simulink model "sysgenQAM16"  (Simulink 7.3)
settings: Solver=ode45  StartTime=0.0  StopTime=5000  RelTol=1e-3
PreLoadFcn:
  | xlrequire('PreLoadFcn')
values from neighbouring files (symbols this model uses):
  hh = hh1/max(hh1)    [sysgenCostasLoop_PreLoadFcn.m]
  j = find(xLabel==')')    [sdspfscope2_r13.m]
  k = (k-1)*3+2    [sdspfscope2_r13.m]
  mu = xfix({xlSigned, 18, 15, xlRound, xlSaturate}, mu)    [lmsErr.m]
undefined symbols (not defined in the file or in its folder): chan, k_i0, k_p0, xlipgetpartsetting, xlsfunxy
libraries: xbsIndex_r4 x263, dspmlti4 x2, dspsigops x2, dspbuff3 x1, xbsCopyrightNotice_r4 x1, dspobslib x1, simulink x1, dspsnks4 x1
(part 2 of 4)

== system sysgenQAM16/Carrier Recovery/DPLL Loop Filter ==
  phs_err : Inport  OutDataType=sfix(16)  OutScaling=2^0
  KI : xbsIndex_r4/Constant  Priority=5  arith_type=Signed (2's comp)  const=k_i0  n_bits=16  bin_pt=15  explicit_period=on  period=4  equ=P=C  opselect=C  inp2=PCIN>>17  opr=+  inp1=P  carry=CIN  dbl_ovrd=off  block_type=constant
      settings: block_version=VER_STRING_GOES_HERE
  KP : xbsIndex_r4/Constant  Priority=5  arith_type=Signed (2's comp)  const=k_p0  n_bits=16  bin_pt=15  explicit_period=on  period=4  equ=P=C  opselect=C  inp2=PCIN>>17  opr=+  inp1=P  carry=CIN  dbl_ovrd=off  block_type=constant
      settings: block_version=VER_STRING_GOES_HERE
  MPY KI : xbsIndex_r4/Mult  precision=User Defined  arith_type="Signed  (2's comp)"  n_bits=32  bin_pt=28  quantization=Truncate  overflow=Wrap  en=off  latency=0  dbl_ovrd=off  use_behavioral_HDL=off  opt=Speed  use_embedded=on  optimum_pipeline=off  pipeline=off  use_rpm=off  placement_style=Rectangular shape  block_type=mult
      settings: infoedit=Multiplies two values.<P><P>Hardware notes: To use the internal pipeline stage of the dedicated multiplier you must select 'Pipeline to Greatest Extent Possible'.  xl_area=[11 0 0 22 0 2 0]  block_version=VER_STRING_GOES_HERE
  MPY KP : xbsIndex_r4/Mult  precision=User Defined  arith_type="Signed  (2's comp)"  n_bits=32  bin_pt=28  quantization=Truncate  overflow=Wrap  en=off  latency=0  dbl_ovrd=off  use_behavioral_HDL=off  opt=Speed  use_embedded=on  optimum_pipeline=off  pipeline=off  use_rpm=off  placement_style=Rectangular shape  block_type=mult
      settings: infoedit=Multiplies two values.<P><P>Hardware notes: To use the internal pipeline stage of the dedicated multiplier you must select 'Pipeline to Greatest Extent Possible'.  xl_area=[11 0 0 22 0 2 0]  block_version=VER_STRING_GOES_HERE
  addsub : xbsIndex_r4/AddSub  mode=Addition  use_carryin=off  use_carryout=off  en=off  latency=0  precision=User Defined  arith_type=Unsigned  n_bits=10  bin_pt=10  quantization=Truncate  overflow=Wrap  dbl_ovrd=off  use_behavioral_HDL=on  hw_selection=Fabric  pipelined=off  use_rpm=off  block_type=addsub
      settings: xl_area=[14 0 0 28 0 0 0]  block_version=VER_STRING_GOES_HERE
  addsub1 : xbsIndex_r4/AddSub  mode=Addition  use_carryin=off  use_carryout=off  en=off  latency=0  precision=User Defined  arith_type="Signed  (2's comp)"  n_bits=32  bin_pt=28  quantization="Round  (unbiased: +/- Inf)"  overflow=Wrap  dbl_ovrd=off  use_behavioral_HDL=on  hw_selection=Fabric  pipelined=off  use_rpm=off  block_type=addsub
      settings: xl_area=[16 0 0 32 0 0 0]  block_version=VER_STRING_GOES_HERE
  register : xbsIndex_r4/Register  init=0  rst=off  en=off  dbl_ovrd=off  block_type=register
      settings: xl_area=[16 32 0 0 0 0 0]  block_version=VER_STRING_GOES_HERE
  y : Outport  OutDataType=sfix(16)  OutScaling=2^0
  wires:
  KI/1 -> MPY KI/2
  KP/1 -> MPY KP/2
  MPY KI/1 -> addsub1/1
  phs_err/1 -> MPY KI/1, MPY KP/1
  register/1 -> addsub1/2
  addsub1/1 -> addsub/2, register/1
  MPY KP/1 -> addsub/1
  addsub/1 -> y/1

== system sysgenQAM16/Carrier Recovery/Phase Detector ==
  note: The slicer circuit consistis primarily of several
      | comparators and a small look-up table.
  note: The arctangent operation is performed using
      | a custom CORDIC processor.
  I_in : Inport  OutDataType=sfix(16)  OutScaling=2^0
  Q_in : Inport  Port=2  OutDataType=sfix(16)  OutScaling=2^0
  Constant : xbsIndex_r4/Constant  arith_type=Signed (2's comp)  const=0  n_bits=1  bin_pt=0  explicit_period=off  period=1  equ=P=C  opselect=C  inp2=PCIN>>17  opr=+  inp1=P  carry=CIN  dbl_ovrd=off  block_type=constant
      settings: block_version=VER_STRING_GOES_HERE
  Cordic : Subsystem
  NegB_Cmplx Mult : Subsystem
  Slicer : Subsystem
  Terminator : Terminator
  Terminator1 : Terminator
  det_I : Outport  OutDataType=sfix(16)  OutScaling=2^0
  det_Q : Outport  Port=2  OutDataType=sfix(16)  OutScaling=2^0
  phs_err : Outport  Port=3  OutDataType=sfix(16)  OutScaling=2^0
  wires:
  NegB_Cmplx Mult/1(p_r) -> Cordic/1(x)
  Cordic/3(z_n) -> phs_err/1
  Constant/1 -> Cordic/3(z)
  Cordic/1(x_n) -> Terminator/1
  Cordic/2(y_n) -> Terminator1/1
  NegB_Cmplx Mult/2(p_i) -> Cordic/2(y)
  Slicer/2(det_Q) -> NegB_Cmplx Mult/2(a_i), det_Q/1
  Slicer/1(det_ I) -> NegB_Cmplx Mult/1(a_r), det_I/1
  Q_in/1 -> Slicer/2(Q_in), NegB_Cmplx Mult/4(b_i)
  I_in/1 -> Slicer/1(I_in), NegB_Cmplx Mult/3(b_r)

== system sysgenQAM16/Channel/Channel ==
  x_n : Inport  OutDataType=sfix(16)  OutScaling=2^0
  Channel Response : Subsystem
  y_n : Outport  OutDataType=sfix(16)  OutScaling=2^0
  wires:
  Channel Response/1(y_n) -> y_n/1
  x_n/1 -> Channel Response/1(x_n)

== system sysgenQAM16/Channel/Channel1 ==
  x_n : Inport  OutDataType=sfix(16)  OutScaling=2^0
  Channel Response : Subsystem
  y_n : Outport  OutDataType=sfix(16)  OutScaling=2^0
  wires:
  Channel Response/1(y_n) -> y_n/1
  x_n/1 -> Channel Response/1(x_n)

== system sysgenQAM16/Doppler/TX Doppler ==
  In1 : Inport  OutDataType=sfix(16)  OutScaling=2^0
  Sum5 : Sum  Inputs=|++  OutDataType=sfix(16)  OutScaling=2^0  SaturateOnIntegerOverflow=on  InputSameDT=on  OutDataTypeStr=Inherit: Same as first input
  Trigonometric Function1 : Trigonometry  Operator=cos
  Trigonometric Function2 : Trigonometry
  Unit Delay2 : UnitDelay
  c2 : Gain  Gain=2*pi  ParameterDataType=sfix(16)  ParameterScaling=2^0  OutDataType=sfix(16)  OutScaling=2^0  SaturateOnIntegerOverflow=on  OutDataTypeStr=Inherit: Same as input  ParamDataTypeStr=Inherit: Same as input
  c3 : Gain  ParameterDataType=sfix(16)  ParameterScaling=2^0  OutDataType=sfix(16)  OutScaling=2^0  SaturateOnIntegerOverflow=on  OutDataTypeStr=Inherit: Same as input  ParamDataTypeStr=Inherit: Same as input
  Cos : Outport  OutDataType=sfix(16)  OutScaling=2^0
  Sin : Outport  Port=2  OutDataType=sfix(16)  OutScaling=2^0
  DDS Theta : Outport  Port=3  OutDataType=sfix(16)  OutScaling=2^0
  wires:
  c2/1 -> Trigonometric Function1/1, Trigonometric Function2/1, DDS Theta/1
  Sum5/1 -> Unit Delay2/1
  Unit Delay2/1 -> c2/1, Sum5/2
  Trigonometric Function2/1 -> c3/1
  c3/1 -> Sin/1
  Trigonometric Function1/1 -> Cos/1
  In1/1 -> Sum5/1

== system sysgenQAM16/16-QAM Data Shaping & Interpolation/QAM16 Source/QAM16 - I ==
  Constant : Constant  Value=3  OutDataType=sfix(16)  OutScaling=2^0
  Gain : Gain  Gain=2  ParameterDataType=sfix(16)  ParameterScaling=2^0  OutDataType=sfix(16)  OutScaling=2^0  SaturateOnIntegerOverflow=on  OutDataTypeStr=Inherit: Same as input  ParamDataTypeStr=Inherit: Same as input
  Gain1 : Gain  Gain=1/3  ParameterDataType=sfix(16)  ParameterScaling=2^0  OutDataType=sfix(16)  OutScaling=2^0  SaturateOnIntegerOverflow=on  OutDataTypeStr=Inherit: Same as input  ParamDataTypeStr=Inherit: Same as input
  Random Integer Generator : Subsystem  mask{M=4, seed=11, Ts=4}
      mask prompts: M "M-ary Number"; seed "Initial seed"; Ts "Sample Time"
  Sum : Sum  Inputs=|+-  OutDataType=sfix(16)  OutScaling=2^0  SaturateOnIntegerOverflow=on  InputSameDT=on  OutDataTypeStr=Inherit: Same as first input
  I : Outport  OutDataType=sfix(16)  OutScaling=2^0
  wires:
  Gain1/1 -> I/1
  Sum/1 -> Gain1/1
  Constant/1 -> Sum/2
  Gain/1 -> Sum/1
  Random Integer Generator/1(Out1) -> Gain/1

== system sysgenQAM16/16-QAM Data Shaping & Interpolation/QAM16 Source/QAM16 -Q ==
  Constant : Constant  Value=3  OutDataType=sfix(16)  OutScaling=2^0
  Gain : Gain  Gain=2  ParameterDataType=sfix(16)  ParameterScaling=2^0  OutDataType=sfix(16)  OutScaling=2^0  SaturateOnIntegerOverflow=on  OutDataTypeStr=Inherit: Same as input  ParamDataTypeStr=Inherit: Same as input
  Gain1 : Gain  Gain=1/3  ParameterDataType=sfix(16)  ParameterScaling=2^0  OutDataType=sfix(16)  OutScaling=2^0  SaturateOnIntegerOverflow=on  OutDataTypeStr=Inherit: Same as input  ParamDataTypeStr=Inherit: Same as input
  Random Integer Generator : Subsystem  mask{M=4, seed=72, Ts=4}
      mask prompts: M "M-ary Number"; seed "Initial seed"; Ts "Sample Time"
  Sum : Sum  Inputs=|+-  OutDataType=sfix(16)  OutScaling=2^0  SaturateOnIntegerOverflow=on  InputSameDT=on  OutDataTypeStr=Inherit: Same as first input
  Q : Outport  OutDataType=sfix(16)  OutScaling=2^0
  wires:
  Gain1/1 -> Q/1
  Sum/1 -> Gain1/1
  Constant/1 -> Sum/2
  Gain/1 -> Sum/1
  Random Integer Generator/1(Out1) -> Gain/1

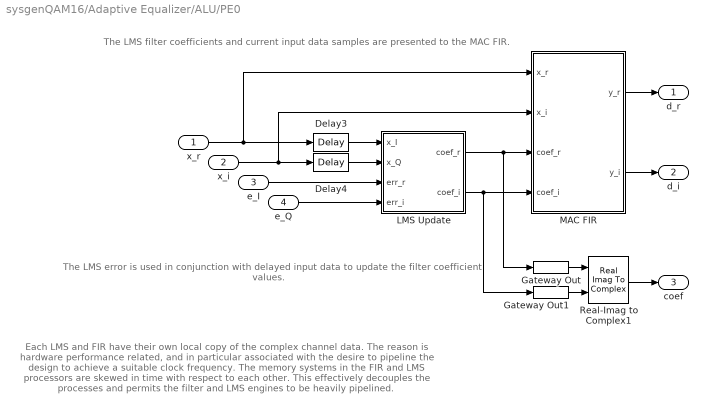
== system sysgenQAM16/Adaptive Equalizer/ALU/PE0 ==
  note: The LMS error is used in conjunction with
      | delayed input data to update the filter
      | coefficient values.
  note: The LMS filter coefficients and current input
      | data samples are presented to the MAC FIR.
  note: Each LMS and FIR have their own local copy of the complex channel data. The reason is hardware
      | performance related, and in particular associated with the desire to pipeline the design to achieve
      | a suitable clock frequency. The memory systems in the FIR and LMS processors are skewed in
      | time with respect to each other. This effectively decouples the processes and permits the filter
      | and LMS engines to be heavily pipelined.
  x_r : Inport  OutDataType=sfix(16)  OutScaling=2^0
  x_i : Inport  Port=2  OutDataType=sfix(16)  OutScaling=2^0
  e_I : Inport  Port=3  OutDataType=sfix(16)  OutScaling=2^0
  e_Q : Inport  Port=4  OutDataType=sfix(16)  OutScaling=2^0
  Delay3 : xbsIndex_r4/Delay  en=off  latency=k  dbl_ovrd=off  reg_retiming=off  block_type=delay
      settings: infoedit="Delay line having  configurable length.<P><P>Hardware notes: A delay line is a chain, each link of which is an SRL16 followed by a flip-flop. If register retiming is enabled, the delay line is a chain of flip-flops."  xl_area=[8 16 0 16 0 0 0]  block_version=VER_STRING_GOES_HERE
  Delay4 : xbsIndex_r4/Delay  en=off  latency=k  dbl_ovrd=off  reg_retiming=off  block_type=delay
      settings: infoedit="Delay line having  configurable length.<P><P>Hardware notes: A delay line is a chain, each link of which is an SRL16 followed by a flip-flop. If register retiming is enabled, the delay line is a chain of flip-flops."  xl_area=[8 16 0 16 0 0 0]  block_version=VER_STRING_GOES_HERE
  Gateway Out : xbsIndex_r4/Gateway Out  hdl_port=off  timing_constraint=None  locs_specified=off  LOCs={}  block_type=gatewayout
      settings: infoedit="Gateway out block.  Converts Xilinx fixed point inputs into ouputs of type Simulink integer, double, or fixed point.<P><P>Hardware notes:  In hardware these blocks become top level output ports or are discarded, depending on how they are configured."  xl_area=[0 0 0 0 0 0 0]  block_version=VER_STRING_GOES_HERE
  Gateway Out1 : xbsIndex_r4/Gateway Out  hdl_port=off  timing_constraint=None  locs_specified=off  LOCs={}  block_type=gatewayout
      settings: infoedit="Gateway out block.  Converts Xilinx fixed point inputs into ouputs of type Simulink integer, double, or fixed point.<P><P>Hardware notes:  In hardware these blocks become top level output ports or are discarded, depending on how they are configured."  xl_area=[0 0 0 0 0 0 0]  block_version=VER_STRING_GOES_HERE
  LMS Update : Subsystem
  MAC FIR : Subsystem
  Real-Imag to Complex1 : RealImagToComplex
  d_r : Outport  OutDataType=sfix(16)  OutScaling=2^0
  d_i : Outport  Port=2  OutDataType=sfix(16)  OutScaling=2^0
  coef : Outport  Port=3  OutDataType=sfix(16)  OutScaling=2^0
  wires:
  x_r/1 -> Delay3/1, MAC FIR/1(x_r)
  x_i/1 -> Delay4/1, MAC FIR/2(x_i)
  e_I/1 -> LMS Update/3(err_r)
  e_Q/1 -> LMS Update/4(err_i)
  Delay3/1 -> LMS Update/1(x_I)
  Delay4/1 -> LMS Update/2(x_Q)
  MAC FIR/1(y_r) -> d_r/1
  MAC FIR/2(y_i) -> d_i/1
  Gateway Out/1 -> Real-Imag to Complex1/1
  Gateway Out1/1 -> Real-Imag to Complex1/2
  Real-Imag to Complex1/1 -> coef/1
  LMS Update/2(coef_i) -> MAC FIR/4(coef_i), Gateway Out1/1
  LMS Update/1(coef_r) -> MAC FIR/3(coef_r), Gateway Out/1

== system sysgenQAM16/Adaptive Equalizer/ALU/PE1 ==
  x_r : Inport  OutDataType=sfix(16)  OutScaling=2^0
  x_i : Inport  Port=2  OutDataType=sfix(16)  OutScaling=2^0
  e_I : Inport  Port=3  OutDataType=sfix(16)  OutScaling=2^0
  e_Q : Inport  Port=4  OutDataType=sfix(16)  OutScaling=2^0
  Delay1 : xbsIndex_r4/Delay  en=off  latency=k  dbl_ovrd=off  reg_retiming=off  block_type=delay
      settings: infoedit="Delay line having  configurable length.<P><P>Hardware notes: A delay line is a chain, each link of which is an SRL16 followed by a flip-flop. If register retiming is enabled, the delay line is a chain of flip-flops."  xl_area=[8 16 0 16 0 0 0]  block_version=VER_STRING_GOES_HERE
  Delay2 : xbsIndex_r4/Delay  en=off  latency=k  dbl_ovrd=off  reg_retiming=off  block_type=delay
      settings: infoedit="Delay line having  configurable length.<P><P>Hardware notes: A delay line is a chain, each link of which is an SRL16 followed by a flip-flop. If register retiming is enabled, the delay line is a chain of flip-flops."  xl_area=[8 16 0 16 0 0 0]  block_version=VER_STRING_GOES_HERE
  Gateway Out2 : xbsIndex_r4/Gateway Out  hdl_port=off  timing_constraint=None  locs_specified=off  LOCs={}  block_type=gatewayout
      settings: infoedit="Gateway out block.  Converts Xilinx fixed point inputs into ouputs of type Simulink integer, double, or fixed point.<P><P>Hardware notes:  In hardware these blocks become top level output ports or are discarded, depending on how they are configured."  xl_area=[0 0 0 0 0 0 0]  block_version=VER_STRING_GOES_HERE
  Gateway Out3 : xbsIndex_r4/Gateway Out  hdl_port=off  timing_constraint=None  locs_specified=off  LOCs={}  block_type=gatewayout
      settings: infoedit="Gateway out block.  Converts Xilinx fixed point inputs into ouputs of type Simulink integer, double, or fixed point.<P><P>Hardware notes:  In hardware these blocks become top level output ports or are discarded, depending on how they are configured."  xl_area=[0 0 0 0 0 0 0]  block_version=VER_STRING_GOES_HERE
  LMS Update : Subsystem
  MAC FIR : Subsystem
  Real-Imag to Complex2 : RealImagToComplex
  d_r : Outport  OutDataType=sfix(16)  OutScaling=2^0
  d_i : Outport  Port=2  OutDataType=sfix(16)  OutScaling=2^0
  coef : Outport  Port=3  OutDataType=sfix(16)  OutScaling=2^0
  wires:
  Gateway Out2/1 -> Real-Imag to Complex2/1
  Gateway Out3/1 -> Real-Imag to Complex2/2
  Real-Imag to Complex2/1 -> coef/1
  Delay2/1 -> LMS Update/2(x_Q)
  Delay1/1 -> LMS Update/1(x_I)
  LMS Update/1(coef_r) -> MAC FIR/3(coef_r), Gateway Out2/1
  LMS Update/2(coef_i) -> MAC FIR/4(coef_i), Gateway Out3/1
  MAC FIR/1(y_r) -> d_r/1
  MAC FIR/2(y_i) -> d_i/1
  e_Q/1 -> LMS Update/4(err_i)
  e_I/1 -> LMS Update/3(err_r)
  x_i/1 -> Delay2/1, MAC FIR/2(x_i)
  x_r/1 -> Delay1/1, MAC FIR/1(x_r)

== system sysgenQAM16/Carrier Recovery/Phase Detector/Cordic ==
  x : Inport  OutDataType=sfix(16)  OutScaling=2^0
  y : Inport  Port=2  OutDataType=sfix(16)  OutScaling=2^0
  z : Inport  Port=3  OutDataType=sfix(16)  OutScaling=2^0
  Cordic Fine Angle PE : Subsystem
  Quadrant  Correct : Subsystem
  Quadrant  Map : Subsystem
  x_n : Outport  OutDataType=sfix(16)  OutScaling=2^0
  y_n : Outport  Port=2  OutDataType=sfix(16)  OutScaling=2^0
  z_n : Outport  Port=3  OutDataType=sfix(16)  OutScaling=2^0
  wires:
  Cordic Fine Angle PE/1(x_n) -> x_n/1
  Cordic Fine Angle PE/2(y_n) -> y_n/1
  Cordic Fine Angle PE/3(z_n) -> Quadrant  Correct/1(z_in)
  y/1 -> Quadrant  Map/2(y)
  x/1 -> Quadrant  Map/1(x)
  Quadrant  Map/2(y_map) -> Cordic Fine Angle PE/2(y_0)
  Quadrant  Map/1(x_map) -> Cordic Fine Angle PE/1(x_0)
  Quadrant  Correct/1(z_out) -> z_n/1
  Quadrant  Map/4(z_mux_sel) -> Quadrant  Correct/3(z_mux_sel)
  Quadrant  Map/3(" PI:2_add:sub") -> Quadrant  Correct/2(pi:2_add:sub)
  z/1 -> Cordic Fine Angle PE/3(z_0)

== system sysgenQAM16/Carrier Recovery/Phase Detector/NegB_Cmplx Mult ==
  a_r : Inport  OutDataType=sfix(16)  OutScaling=2^0
  a_i : Inport  Port=2  OutDataType=sfix(16)  OutScaling=2^0
  b_r : Inport  Port=3  OutDataType=sfix(16)  OutScaling=2^0
  b_i : Inport  Port=4  OutDataType=sfix(16)  OutScaling=2^0
  AddSub : xbsIndex_r4/AddSub  mode=Addition  use_carryin=off  use_carryout=off  en=off  latency=0  precision=User Defined  arith_type="Signed  (2's comp)"  n_bits=lms_mult_post_add_ni  bin_pt=lms_mult_post_add_nf  quantization=Truncate  overflow=Wrap  dbl_ovrd=off  use_behavioral_HDL=on  hw_selection=Fabric  pipelined=off  use_rpm=on  block_type=addsub
      settings: xl_area=[18 0 0 36 0 0 0]  block_version=VER_STRING_GOES_HERE
  AddSub1 : xbsIndex_r4/AddSub  mode=Subtraction  use_carryin=off  use_carryout=off  en=off  latency=0  precision=User Defined  arith_type="Signed  (2's comp)"  n_bits=lms_mult_post_add_ni  bin_pt=lms_mult_post_add_nf  quantization=Truncate  overflow=Wrap  dbl_ovrd=off  use_behavioral_HDL=on  hw_selection=Fabric  pipelined=off  use_rpm=on  block_type=addsub
      settings: xl_area=[18 0 0 36 0 0 0]  block_version=VER_STRING_GOES_HERE
  Mult{1..4} (4 alike) : xbsIndex_r4/Mult  precision=User Defined  arith_type="Signed  (2's comp)"  n_bits=lms_mult_ni  bin_pt=lms_mult_nf  quantization=Truncate  overflow=Wrap  en=off  latency=0  dbl_ovrd=off  use_behavioral_HDL=off  opt=Speed  use_embedded=on  optimum_pipeline=off  pipeline=off  use_rpm=on  placement_style=Rectangular shape  block_type=mult
      settings: infoedit=Multiplies two values.<P><P>Hardware notes: To use the internal pipeline stage of the dedicated multiplier you must select 'Pipeline to Greatest Extent Possible'.  xl_area=[69 0 0 136 0 3 0]  block_version=VER_STRING_GOES_HERE
  p_r : Outport  OutDataType=sfix(16)  OutScaling=2^0
  p_i : Outport  Port=2  OutDataType=sfix(16)  OutScaling=2^0
  wires:
  Mult4/1 -> AddSub/1
  a_i/1 -> Mult1/1, Mult3/2
  b_r/1 -> Mult4/2, Mult3/1
  b_i/1 -> Mult1/2, Mult2/2
  a_r/1 -> Mult4/1, Mult2/1
  Mult1/1 -> AddSub/2
  Mult2/1 -> AddSub1/1
  Mult3/1 -> AddSub1/2
  AddSub/1 -> p_r/1
  AddSub1/1 -> p_i/1

== system sysgenQAM16/Carrier Recovery/Phase Detector/Slicer ==
  I_in : Inport  OutDataType=sfix(16)  OutScaling=2^0
  Q_in : Inport  Port=2  OutDataType=sfix(16)  OutScaling=2^0
  I Map : Subsystem
  Q Map : Subsystem
  det_ I : Outport  OutDataType=sfix(16)  OutScaling=2^0
  det_Q : Outport  Port=2  OutDataType=sfix(16)  OutScaling=2^0
  wires:
  Q Map/1(det) -> det_Q/1
  I Map/1(det) -> det_ I/1
  I_in/1 -> I Map/1(x_n)
  Q_in/1 -> Q Map/1(x_n)

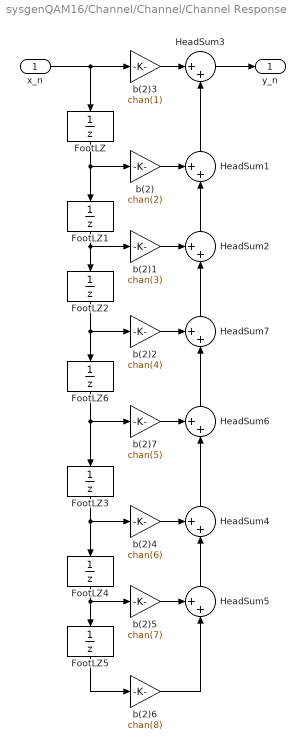
== system sysgenQAM16/Channel/Channel/Channel Response ==
  x_n : Inport  OutDataType=sfix(16)  OutScaling=2^0
  FootLZ : UnitDelay
  FootLZ{1..2,4..6} (5 alike) : UnitDelay  SampleTime=-1
  FootLZ3 : UnitDelay
  HeadSum{1..2,4..7} (6 alike) : Sum  Inputs=++|  OutDataType=sfix(16)  OutScaling=2^0  SaturateOnIntegerOverflow=on  InputSameDT=on  OutDataTypeStr=Inherit: Same as first input
  HeadSum3 : Sum  Inputs=|++  OutDataType=sfix(16)  OutScaling=2^0  SaturateOnIntegerOverflow=on  InputSameDT=on  OutDataTypeStr=Inherit: Same as first input
  b(2) : Gain  Gain=chan(2)  ParameterDataType=sfix(16)  ParameterScaling=2^0  OutDataType=sfix(16)  OutScaling=2^0  SaturateOnIntegerOverflow=on  OutDataTypeStr=Inherit: Same as input  ParamDataTypeStr=Inherit: Same as input
  b(2)1 : Gain  Gain=chan(3)  ParameterDataType=sfix(16)  ParameterScaling=2^0  OutDataType=sfix(16)  OutScaling=2^0  SaturateOnIntegerOverflow=on  OutDataTypeStr=Inherit: Same as input  ParamDataTypeStr=Inherit: Same as input
  b(2)2 : Gain  Gain=chan(4)  ParameterDataType=sfix(16)  ParameterScaling=2^0  OutDataType=sfix(16)  OutScaling=2^0  SaturateOnIntegerOverflow=on  OutDataTypeStr=Inherit: Same as input  ParamDataTypeStr=Inherit: Same as input
  b(2)3 : Gain  Gain=chan(1)  ParameterDataType=sfix(16)  ParameterScaling=2^0  OutDataType=sfix(16)  OutScaling=2^0  SaturateOnIntegerOverflow=on  OutDataTypeStr=Inherit: Same as input  ParamDataTypeStr=Inherit: Same as input
  b(2)4 : Gain  Gain=chan(6)  ParameterDataType=sfix(16)  ParameterScaling=2^0  OutDataType=sfix(16)  OutScaling=2^0  SaturateOnIntegerOverflow=on  OutDataTypeStr=Inherit: Same as input  ParamDataTypeStr=Inherit: Same as input
  b(2)5 : Gain  Gain=chan(7)  ParameterDataType=sfix(16)  ParameterScaling=2^0  OutDataType=sfix(16)  OutScaling=2^0  SaturateOnIntegerOverflow=on  OutDataTypeStr=Inherit: Same as input  ParamDataTypeStr=Inherit: Same as input
  b(2)6 : Gain  Gain=chan(8)  ParameterDataType=sfix(16)  ParameterScaling=2^0  OutDataType=sfix(16)  OutScaling=2^0  SaturateOnIntegerOverflow=on  OutDataTypeStr=Inherit: Same as input  ParamDataTypeStr=Inherit: Same as input
  b(2)7 : Gain  Gain=chan(5)  ParameterDataType=sfix(16)  ParameterScaling=2^0  OutDataType=sfix(16)  OutScaling=2^0  SaturateOnIntegerOverflow=on  OutDataTypeStr=Inherit: Same as input  ParamDataTypeStr=Inherit: Same as input
  y_n : Outport  OutDataType=sfix(16)  OutScaling=2^0
  wires:
  HeadSum3/1 -> y_n/1
  HeadSum1/1 -> HeadSum3/2
  b(2)3/1 -> HeadSum3/1
  x_n/1 -> b(2)3/1, FootLZ/1
  HeadSum2/1 -> HeadSum1/2
  b(2)1/1 -> HeadSum2/1
  b(2)/1 -> HeadSum1/1
  FootLZ1/1 -> b(2)1/1, FootLZ2/1
  FootLZ/1 -> FootLZ1/1, b(2)/1
  FootLZ2/1 -> b(2)2/1, FootLZ6/1
  b(2)7/1 -> HeadSum6/1
  b(2)6/1 -> HeadSum5/2
  HeadSum5/1 -> HeadSum4/2
  b(2)5/1 -> HeadSum5/1
  b(2)4/1 -> HeadSum4/1
  FootLZ5/1 -> b(2)6/1
  FootLZ4/1 -> b(2)5/1, FootLZ5/1
  FootLZ3/1 -> FootLZ4/1, b(2)4/1
  FootLZ6/1 -> b(2)7/1, FootLZ3/1
  b(2)2/1 -> HeadSum7/1
  HeadSum7/1 -> HeadSum2/2
  HeadSum4/1 -> HeadSum6/2
  HeadSum6/1 -> HeadSum7/2

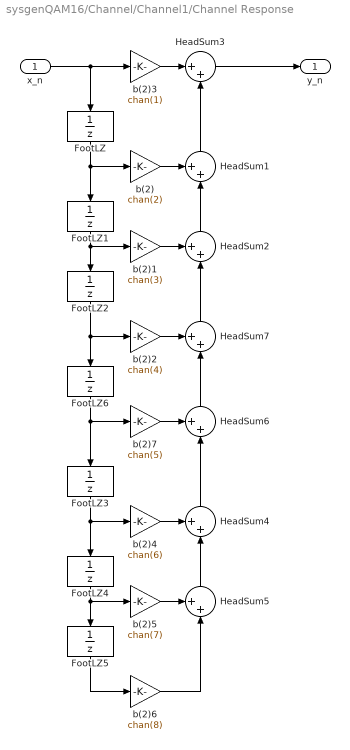
== system sysgenQAM16/Channel/Channel1/Channel Response ==
  x_n : Inport  OutDataType=sfix(16)  OutScaling=2^0
  FootLZ : UnitDelay
  FootLZ{1..2,4..6} (5 alike) : UnitDelay  SampleTime=-1
  FootLZ3 : UnitDelay
  HeadSum{1..2,4..7} (6 alike) : Sum  Inputs=++|  OutDataType=sfix(16)  OutScaling=2^0  SaturateOnIntegerOverflow=on  InputSameDT=on  OutDataTypeStr=Inherit: Same as first input
  HeadSum3 : Sum  Inputs=|++  OutDataType=sfix(16)  OutScaling=2^0  SaturateOnIntegerOverflow=on  InputSameDT=on  OutDataTypeStr=Inherit: Same as first input
  b(2) : Gain  Gain=chan(2)  ParameterDataType=sfix(16)  ParameterScaling=2^0  OutDataType=sfix(16)  OutScaling=2^0  SaturateOnIntegerOverflow=on  OutDataTypeStr=Inherit: Same as input  ParamDataTypeStr=Inherit: Same as input
  b(2)1 : Gain  Gain=chan(3)  ParameterDataType=sfix(16)  ParameterScaling=2^0  OutDataType=sfix(16)  OutScaling=2^0  SaturateOnIntegerOverflow=on  OutDataTypeStr=Inherit: Same as input  ParamDataTypeStr=Inherit: Same as input
  b(2)2 : Gain  Gain=chan(4)  ParameterDataType=sfix(16)  ParameterScaling=2^0  OutDataType=sfix(16)  OutScaling=2^0  SaturateOnIntegerOverflow=on  OutDataTypeStr=Inherit: Same as input  ParamDataTypeStr=Inherit: Same as input
  b(2)3 : Gain  Gain=chan(1)  ParameterDataType=sfix(16)  ParameterScaling=2^0  OutDataType=sfix(16)  OutScaling=2^0  SaturateOnIntegerOverflow=on  OutDataTypeStr=Inherit: Same as input  ParamDataTypeStr=Inherit: Same as input
  b(2)4 : Gain  Gain=chan(6)  ParameterDataType=sfix(16)  ParameterScaling=2^0  OutDataType=sfix(16)  OutScaling=2^0  SaturateOnIntegerOverflow=on  OutDataTypeStr=Inherit: Same as input  ParamDataTypeStr=Inherit: Same as input
  b(2)5 : Gain  Gain=chan(7)  ParameterDataType=sfix(16)  ParameterScaling=2^0  OutDataType=sfix(16)  OutScaling=2^0  SaturateOnIntegerOverflow=on  OutDataTypeStr=Inherit: Same as input  ParamDataTypeStr=Inherit: Same as input
  b(2)6 : Gain  Gain=chan(8)  ParameterDataType=sfix(16)  ParameterScaling=2^0  OutDataType=sfix(16)  OutScaling=2^0  SaturateOnIntegerOverflow=on  OutDataTypeStr=Inherit: Same as input  ParamDataTypeStr=Inherit: Same as input
  b(2)7 : Gain  Gain=chan(5)  ParameterDataType=sfix(16)  ParameterScaling=2^0  OutDataType=sfix(16)  OutScaling=2^0  SaturateOnIntegerOverflow=on  OutDataTypeStr=Inherit: Same as input  ParamDataTypeStr=Inherit: Same as input
  y_n : Outport  OutDataType=sfix(16)  OutScaling=2^0
  wires:
  HeadSum3/1 -> y_n/1
  HeadSum1/1 -> HeadSum3/2
  b(2)3/1 -> HeadSum3/1
  x_n/1 -> b(2)3/1, FootLZ/1
  HeadSum2/1 -> HeadSum1/2
  b(2)1/1 -> HeadSum2/1
  b(2)/1 -> HeadSum1/1
  FootLZ1/1 -> b(2)1/1, FootLZ2/1
  FootLZ/1 -> FootLZ1/1, b(2)/1
  HeadSum4/1 -> HeadSum6/2
  b(2)7/1 -> HeadSum6/1
  b(2)6/1 -> HeadSum5/2
  HeadSum5/1 -> HeadSum4/2
  b(2)5/1 -> HeadSum5/1
  b(2)4/1 -> HeadSum4/1
  FootLZ5/1 -> b(2)6/1
  FootLZ4/1 -> b(2)5/1, FootLZ5/1
  FootLZ3/1 -> FootLZ4/1, b(2)4/1
  FootLZ2/1 -> b(2)2/1, FootLZ6/1
  FootLZ6/1 -> FootLZ3/1, b(2)7/1
  HeadSum6/1 -> HeadSum7/2
  HeadSum7/1 -> HeadSum2/2
  b(2)2/1 -> HeadSum7/1

== system sysgenQAM16/16-QAM Data Shaping & Interpolation/QAM16 Source/QAM16 - I/Random Integer Generator ==
  Rounding Function : Rounding  Operator=round
  Uniform Random Number : UniformRandomNumber  Minimum=-0.49  Maximum=M-1 + 0.49  Seed=seed  SampleTime=Ts
  Out1 : Outport  OutDataType=sfix(16)  OutScaling=2^0
  wires:
  Uniform Random Number/1 -> Rounding Function/1
  Rounding Function/1 -> Out1/1

== system sysgenQAM16/16-QAM Data Shaping & Interpolation/QAM16 Source/QAM16 -Q/Random Integer Generator ==
  Rounding Function : Rounding  Operator=round
  Uniform Random Number : UniformRandomNumber  Minimum=-0.49  Maximum=M-1 + 0.49  Seed=seed  SampleTime=Ts
  Out1 : Outport  OutDataType=sfix(16)  OutScaling=2^0
  wires:
  Uniform Random Number/1 -> Rounding Function/1
  Rounding Function/1 -> Out1/1

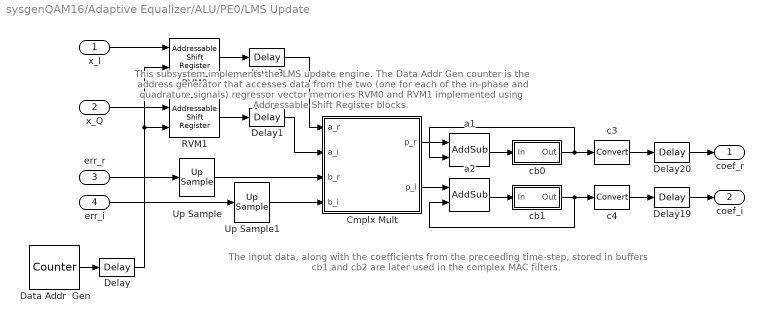
== system sysgenQAM16/Adaptive Equalizer/ALU/PE0/LMS Update ==
  note: This subsystem implements the LMS update engine. The Data Addr Gen
      | counter is the address generator that accesses data from the two (one for each of the
      | in-phase and quadrature signals) regressor vector memories RVM0 and RVM1
      | implemented using Addressable Shift Register blocks.
  note: The input data, along with the coefficients from the
      | preceeding time-step, stored in buffers cb1 and cb2
      | are later used in the complex MAC filters.
  x_I : Inport  OutDataType=sfix(16)  OutScaling=2^0
  x_Q : Inport  Port=2  OutDataType=sfix(16)  OutScaling=2^0
  err_r : Inport  Port=3  OutDataType=sfix(16)  OutScaling=2^0
  err_i : Inport  Port=4  OutDataType=sfix(16)  OutScaling=2^0
  Cmplx Mult : Subsystem
  Data Addr  Gen : xbsIndex_r4/Counter  cnt_type=Count Limited  cnt_to=3  operation=Up  start_count=0  cnt_by_val=1  arith_type=Unsigned  n_bits=2  bin_pt=0  load_pin=off  rst=off  en=off  explicit_period=off  period=T  dbl_ovrd=off  use_behavioral_HDL=off  implementation=Fabric  use_rpm=off  block_type=counter
      settings: infoedit="Configurable up, down and up/down counter.<P><P>Hardware notes: Free running counters are the least expensive in hardware.  A count limited counter is implemented by combining a counter with a comparator."  xl_area=[2 2 0 3 0 0 0]  block_version=VER_STRING_GOES_HERE
  Delay : xbsIndex_r4/Delay  en=off  latency=1  dbl_ovrd=off  reg_retiming=off  block_type=delay
      settings: infoedit="Delay line having  configurable length.<P><P>Hardware notes: A delay line is a chain, each link of which is an SRL16 followed by a flip-flop. If register retiming is enabled, the delay line is a chain of flip-flops."  xl_area=[1 2 0 0 0 0 0]  block_version=VER_STRING_GOES_HERE
  Delay1 : xbsIndex_r4/Delay  en=off  latency=3  dbl_ovrd=off  reg_retiming=off  block_type=delay
      settings: infoedit="Delay line having  configurable length.<P><P>Hardware notes: A delay line is a chain, each link of which is an SRL16 followed by a flip-flop. If register retiming is enabled, the delay line is a chain of flip-flops."  xl_area=[8 16 0 16 0 0 0]  block_version=VER_STRING_GOES_HERE
  Delay19 : xbsIndex_r4/Delay  en=off  latency=6  dbl_ovrd=off  reg_retiming=off  block_type=delay
      settings: infoedit="Delay line having  configurable length.<P><P>Hardware notes: A delay line is a chain, each link of which is an SRL16 followed by a flip-flop. If register retiming is enabled, the delay line is a chain of flip-flops."  xl_area=[9 18 0 18 0 0 0]  block_version=VER_STRING_GOES_HERE
  Delay20 : xbsIndex_r4/Delay  en=off  latency=6  dbl_ovrd=off  reg_retiming=off  block_type=delay
      settings: infoedit="Delay line having  configurable length.<P><P>Hardware notes: A delay line is a chain, each link of which is an SRL16 followed by a flip-flop. If register retiming is enabled, the delay line is a chain of flip-flops."  xl_area=[9 18 0 18 0 0 0]  block_version=VER_STRING_GOES_HERE
  Delay3 : xbsIndex_r4/Delay  en=off  latency=3  dbl_ovrd=off  reg_retiming=off  block_type=delay
      settings: infoedit="Delay line having  configurable length.<P><P>Hardware notes: A delay line is a chain, each link of which is an SRL16 followed by a flip-flop. If register retiming is enabled, the delay line is a chain of flip-flops."  xl_area=[8 16 0 16 0 0 0]  block_version=VER_STRING_GOES_HERE
  RVM0 : xbsIndex_r4/Addressable Shift Register  infer_latency=off  depth=4  initVector=[0]  en=off  dbl_ovrd=off  use_behavioral_HDL=off  use_rpm=off  block_type=addrsr
      settings: infoedit="Delay of configurable length.  Any element in the delay line can be addressed and driven onto the output port.<P><P>Hardware notes: Implemented using SRL16s.  If a Virtex-II device is used, multiple SRLC16s are cascaded together."  xl_area=[8 0 0 16 0 0 0]  block_version=VER_STRING_GOES_HERE
  RVM1 : xbsIndex_r4/Addressable Shift Register  infer_latency=off  depth=4  initVector=[0]  en=off  dbl_ovrd=off  use_behavioral_HDL=off  use_rpm=off  block_type=addrsr
      settings: infoedit="Delay of configurable length.  Any element in the delay line can be addressed and driven onto the output port.<P><P>Hardware notes: Implemented using SRL16s.  If a Virtex-II device is used, multiple SRLC16s are cascaded together."  xl_area=[8 0 0 16 0 0 0]  block_version=VER_STRING_GOES_HERE
  Up Sample : xbsIndex_r4/Up Sample  sample_ratio=4  copy_samples=on  en=off  latency=0  dbl_ovrd=off  block_type=usamp
      settings: infoedit="Up samples input data.  Inserted values  can be zeros or copies of the most recent input sample.<P><P>Hardware notes: No hardware is needed if inserted values are copies of the input sample; otherwise, a mux and single bit flip-flop are used."  xl_area=[0 0 0 0 0 0 0]  block_version=VER_STRING_GOES_HERE
  Up Sample1 : xbsIndex_r4/Up Sample  sample_ratio=4  copy_samples=on  en=off  latency=0  dbl_ovrd=off  block_type=usamp
      settings: infoedit="Up samples input data.  Inserted values  can be zeros or copies of the most recent input sample.<P><P>Hardware notes: No hardware is needed if inserted values are copies of the input sample; otherwise, a mux and single bit flip-flop are used."  xl_area=[0 0 0 0 0 0 0]  block_version=VER_STRING_GOES_HERE
  a1 : xbsIndex_r4/AddSub  mode=Addition  use_carryin=off  use_carryout=off  en=off  latency=0  precision=User Defined  arith_type="Signed  (2's comp)"  n_bits=lms_acc_ni  bin_pt=lms_acc_nf  quantization="Round  (unbiased: +/- Inf)"  overflow=Wrap  dbl_ovrd=off  use_behavioral_HDL=on  hw_selection=Fabric  pipelined=off  use_rpm=on  block_type=addsub
      settings: xl_area=[18 0 0 36 0 0 0]  block_version=VER_STRING_GOES_HERE
  a2 : xbsIndex_r4/AddSub  mode=Addition  use_carryin=off  use_carryout=off  en=off  latency=0  precision=User Defined  arith_type="Signed  (2's comp)"  n_bits=lms_acc_ni  bin_pt=lms_acc_nf  quantization="Round  (unbiased: +/- Inf)"  overflow=Wrap  dbl_ovrd=off  use_behavioral_HDL=on  hw_selection=Fabric  pipelined=off  use_rpm=on  block_type=addsub
      settings: xl_area=[18 0 0 36 0 0 0]  block_version=VER_STRING_GOES_HERE
  c3 : xbsIndex_r4/Convert  arith_type="Signed  (2's comp)"  n_bits=coeff_ni  bin_pt=coeff_nf  quantization="Round  (unbiased: +/- Inf)"  overflow=Wrap  latency=0  dbl_ovrd=off  pipeline=off  block_type=convert
      settings: infoedit=The input is presented at the output after quantization and overflow effects.<P><P>Hardware notes: Additional hardware is used when rounding or saturation is selected and output width is less than the input width.  xl_area=[11 0 0 22 0 0 0]  block_version=VER_STRING_GOES_HERE
  c4 : xbsIndex_r4/Convert  arith_type="Signed  (2's comp)"  n_bits=coeff_ni  bin_pt=coeff_nf  quantization="Round  (unbiased: +/- Inf)"  overflow=Wrap  latency=0  dbl_ovrd=off  pipeline=off  block_type=convert
      settings: infoedit=The input is presented at the output after quantization and overflow effects.<P><P>Hardware notes: Additional hardware is used when rounding or saturation is selected and output width is less than the input width.  xl_area=[11 0 0 22 0 0 0]  block_version=VER_STRING_GOES_HERE
  cb0 : Subsystem
  cb1 : Subsystem
  coef_r : Outport  OutDataType=sfix(16)  OutScaling=2^0
  coef_i : Outport  Port=2  OutDataType=sfix(16)  OutScaling=2^0
  wires:
  x_I/1 -> RVM0/1
  RVM0/1 -> Delay3/1
  x_Q/1 -> RVM1/1
  RVM1/1 -> Delay1/1
  Delay3/1 -> Cmplx Mult/1(a_r)
  Delay1/1 -> Cmplx Mult/2(a_i)
  a1/1 -> cb0/1(In)
  a2/1 -> cb1/1(In)
  cb0/1(Out) -> c3/1, a1/2
  cb1/1(Out) -> c4/1, a2/2
  err_r/1 -> Up Sample/1
  err_i/1 -> Up Sample1/1
  Up Sample/1 -> Cmplx Mult/3(b_r)
  Up Sample1/1 -> Cmplx Mult/4(b_i)
  Data Addr  Gen/1 -> Delay/1
  Delay/1 -> RVM1/2, RVM0/2
  c3/1 -> Delay20/1
  c4/1 -> Delay19/1
  Delay19/1 -> coef_i/1
  Delay20/1 -> coef_r/1
  Cmplx Mult/1(p_r) -> a1/1
  Cmplx Mult/2(p_i) -> a2/1

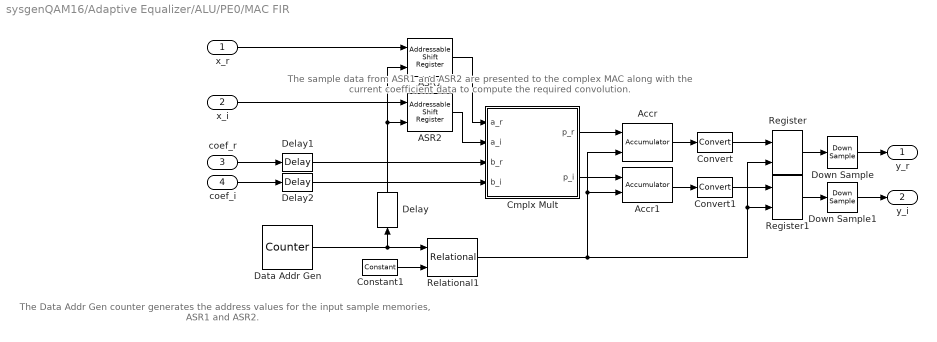
== system sysgenQAM16/Adaptive Equalizer/ALU/PE0/MAC FIR ==
  note: The sample data from ASR1 and ASR2 are presented to the
      | complex MAC along with the current coefficient  data to compute
      | the required convolution.
  note: The Data Addr Gen counter generates the address values for
      | the input sample memories, ASR1 and ASR2.
  x_r : Inport  OutDataType=sfix(16)  OutScaling=2^0
  x_i : Inport  Port=2  OutDataType=sfix(16)  OutScaling=2^0
  coef_r : Inport  Port=3  OutDataType=sfix(16)  OutScaling=2^0
  coef_i : Inport  Port=4  OutDataType=sfix(16)  OutScaling=2^0
  ASR1 : xbsIndex_r4/Addressable Shift Register  infer_latency=off  depth=4  initVector=[0]  en=off  dbl_ovrd=off  use_behavioral_HDL=off  use_rpm=off  block_type=addrsr
      settings: infoedit="Delay of configurable length.  Any element in the delay line can be addressed and driven onto the output port.<P><P>Hardware notes: Implemented using SRL16s.  If a Virtex-II device is used, multiple SRLC16s are cascaded together."  xl_area=[8 0 0 16 0 0 0]  block_version=VER_STRING_GOES_HERE
  ASR2 : xbsIndex_r4/Addressable Shift Register  infer_latency=off  depth=4  initVector=[0]  en=off  dbl_ovrd=off  use_behavioral_HDL=off  use_rpm=off  block_type=addrsr
      settings: infoedit="Delay of configurable length.  Any element in the delay line can be addressed and driven onto the output port.<P><P>Hardware notes: Implemented using SRL16s.  If a Virtex-II device is used, multiple SRLC16s are cascaded together."  xl_area=[8 0 0 16 0 0 0]  block_version=VER_STRING_GOES_HERE
  Accr : xbsIndex_r4/Accumulator  operation=Add  n_bits=46  overflow=Wrap  scale=1  rst=on  hasbypass=on  en=off  dbl_ovrd=off  use_behavioral_HDL=on  implementation=Fabric  block_type=accum
      settings: infoedit="Adder or subtractor-based accumulator.   Output type and binary point position match the input.<P><P>Hardware notes: When \"Reinitialize with Input 'b' on Reset\" is selected, the accumulator is forced to run at the system rate even if the input 'b' is running at a slower rate."  xl_area=[23 46 0 41 0 0 0]  block_version=VER_STRING_GOES_HERE
  Accr1 : xbsIndex_r4/Accumulator  operation=Add  n_bits=46  overflow=Wrap  scale=1  rst=on  hasbypass=on  en=off  dbl_ovrd=off  use_behavioral_HDL=on  implementation=Fabric  block_type=accum
      settings: infoedit="Adder or subtractor-based accumulator.   Output type and binary point position match the input.<P><P>Hardware notes: When \"Reinitialize with Input 'b' on Reset\" is selected, the accumulator is forced to run at the system rate even if the input 'b' is running at a slower rate."  xl_area=[23 46 0 41 0 0 0]  block_version=VER_STRING_GOES_HERE
  Cmplx Mult : Subsystem
  Constant1 : xbsIndex_r4/Constant  arith_type=Unsigned  const=0  n_bits=1  bin_pt=0  explicit_period=on  period=T  equ=P=C  opselect=C  inp2=PCIN>>17  opr=+  inp1=P  carry=CIN  dbl_ovrd=off  block_type=constant
      settings: block_version=VER_STRING_GOES_HERE
  Convert : xbsIndex_r4/Convert  arith_type="Signed  (2's comp)"  n_bits=24  bin_pt=20  quantization="Round  (unbiased: +/- Inf)"  overflow=Wrap  latency=0  dbl_ovrd=off  pipeline=off  block_type=convert
      settings: infoedit=The input is presented at the output after quantization and overflow effects.<P><P>Hardware notes: Additional hardware is used when rounding or saturation is selected and output width is less than the input width.  xl_area=[14 0 0 27 0 0 0]  block_version=VER_STRING_GOES_HERE
  Convert1 : xbsIndex_r4/Convert  arith_type="Signed  (2's comp)"  n_bits=24  bin_pt=20  quantization="Round  (unbiased: +/- Inf)"  overflow=Wrap  latency=0  dbl_ovrd=off  pipeline=off  block_type=convert
      settings: infoedit=The input is presented at the output after quantization and overflow effects.<P><P>Hardware notes: Additional hardware is used when rounding or saturation is selected and output width is less than the input width.  xl_area=[14 0 0 27 0 0 0]  block_version=VER_STRING_GOES_HERE
  Data Addr Gen : xbsIndex_r4/Counter  cnt_type=Count Limited  cnt_to=3  operation=Up  start_count=0  cnt_by_val=1  arith_type=Unsigned  n_bits=2  bin_pt=0  load_pin=off  rst=off  en=off  explicit_period=off  period=T  dbl_ovrd=off  use_behavioral_HDL=off  implementation=Fabric  use_rpm=off  block_type=counter
      settings: infoedit="Configurable up, down and up/down counter.<P><P>Hardware notes: Free running counters are the least expensive in hardware.  A count limited counter is implemented by combining a counter with a comparator."  xl_area=[2 2 0 3 0 0 0]  block_version=VER_STRING_GOES_HERE
  Delay : xbsIndex_r4/Delay  en=off  latency=1  dbl_ovrd=off  reg_retiming=off  block_type=delay
      settings: infoedit="Delay line having  configurable length.<P><P>Hardware notes: A delay line is a chain, each link of which is an SRL16 followed by a flip-flop. If register retiming is enabled, the delay line is a chain of flip-flops."  xl_area=[1 2 0 0 0 0 0]  block_version=VER_STRING_GOES_HERE
  Delay1 : xbsIndex_r4/Delay  en=off  latency=1  dbl_ovrd=off  reg_retiming=off  block_type=delay
      settings: infoedit="Delay line having  configurable length.<P><P>Hardware notes: A delay line is a chain, each link of which is an SRL16 followed by a flip-flop. If register retiming is enabled, the delay line is a chain of flip-flops."  xl_area=[9 18 0 0 0 0 0]  block_version=VER_STRING_GOES_HERE
  Delay2 : xbsIndex_r4/Delay  en=off  latency=1  dbl_ovrd=off  reg_retiming=off  block_type=delay
      settings: infoedit="Delay line having  configurable length.<P><P>Hardware notes: A delay line is a chain, each link of which is an SRL16 followed by a flip-flop. If register retiming is enabled, the delay line is a chain of flip-flops."  xl_area=[9 18 0 0 0 0 0]  block_version=VER_STRING_GOES_HERE
  Down Sample : xbsIndex_r4/Down Sample  sample_ratio=4  sample_phase="Last Value of Frame  (most efficient)"  en=off  latency=1  dbl_ovrd=off  block_type=dsamp
      settings: xl_area=[12 24 0 0 0 0 0]  block_version=VER_STRING_GOES_HERE
  Down Sample1 : xbsIndex_r4/Down Sample  sample_ratio=4  sample_phase="Last Value of Frame  (most efficient)"  en=off  latency=1  dbl_ovrd=off  block_type=dsamp
      settings: xl_area=[12 24 0 0 0 0 0]  block_version=VER_STRING_GOES_HERE
  Register : xbsIndex_r4/Register  init=0  rst=off  en=on  dbl_ovrd=off  block_type=register
      settings: xl_area=[12 24 0 0 0 0 0]  block_version=VER_STRING_GOES_HERE
  Register1 : xbsIndex_r4/Register  init=0  rst=off  en=on  dbl_ovrd=off  block_type=register
      settings: xl_area=[12 24 0 0 0 0 0]  block_version=VER_STRING_GOES_HERE
  Relational1 : xbsIndex_r4/Relational  mode=a=b  en=off  latency=7  dbl_ovrd=off  block_type=relational
      settings: xl_area=[1 2 0 2 0 0 0]  block_version=VER_STRING_GOES_HERE
  y_r : Outport  OutDataType=sfix(16)  OutScaling=2^0
  y_i : Outport  Port=2  OutDataType=sfix(16)  OutScaling=2^0
  wires:
  Delay/1 -> ASR1/2, ASR2/2
  x_r/1 -> ASR1/1
  ASR1/1 -> Cmplx Mult/1(a_r)
  x_i/1 -> ASR2/1
  ASR2/1 -> Cmplx Mult/2(a_i)
  coef_r/1 -> Delay1/1
  coef_i/1 -> Delay2/1
  Delay2/1 -> Cmplx Mult/4(b_i)
  Delay1/1 -> Cmplx Mult/3(b_r)
  Accr/1 -> Convert/1
  Cmplx Mult/1(p_r) -> Accr/1
  Cmplx Mult/2(p_i) -> Accr1/1
  Accr1/1 -> Convert1/1
  Relational1/1 -> Accr/2, Accr1/2, Register/2, Register1/2
  Register/1 -> Down Sample/1
  Register1/1 -> Down Sample1/1
  Convert/1 -> Register/1
  Convert1/1 -> Register1/1
  Down Sample/1 -> y_r/1
  Down Sample1/1 -> y_i/1
  Data Addr Gen/1 -> Relational1/1, Delay/1
  Constant1/1 -> Relational1/2

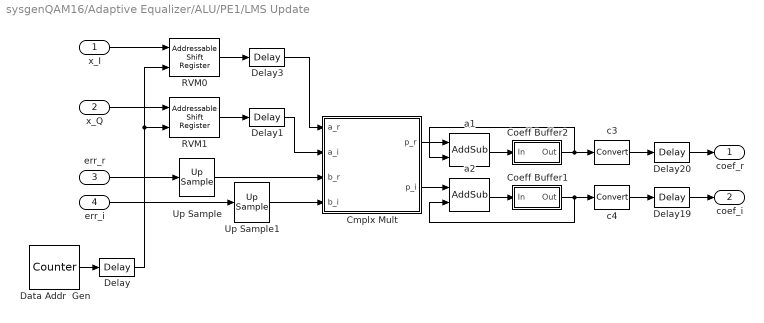
== system sysgenQAM16/Adaptive Equalizer/ALU/PE1/LMS Update ==
  x_I : Inport  OutDataType=sfix(16)  OutScaling=2^0
  x_Q : Inport  Port=2  OutDataType=sfix(16)  OutScaling=2^0
  err_r : Inport  Port=3  OutDataType=sfix(16)  OutScaling=2^0
  err_i : Inport  Port=4  OutDataType=sfix(16)  OutScaling=2^0
  Cmplx Mult : Subsystem
  Coeff Buffer1 : Subsystem
  Coeff Buffer2 : Subsystem
  Data Addr  Gen : xbsIndex_r4/Counter  cnt_type=Count Limited  cnt_to=3  operation=Up  start_count=0  cnt_by_val=1  arith_type=Unsigned  n_bits=2  bin_pt=0  load_pin=off  rst=off  en=off  explicit_period=off  period=T  dbl_ovrd=off  use_behavioral_HDL=off  implementation=Fabric  use_rpm=off  block_type=counter
      settings: infoedit="Configurable up, down and up/down counter.<P><P>Hardware notes: Free running counters are the least expensive in hardware.  A count limited counter is implemented by combining a counter with a comparator."  xl_area=[2 2 0 3 0 0 0]  block_version=VER_STRING_GOES_HERE
  Delay : xbsIndex_r4/Delay  en=off  latency=1  dbl_ovrd=off  reg_retiming=off  block_type=delay
      settings: infoedit="Delay line having  configurable length.<P><P>Hardware notes: A delay line is a chain, each link of which is an SRL16 followed by a flip-flop. If register retiming is enabled, the delay line is a chain of flip-flops."  xl_area=[1 2 0 0 0 0 0]  block_version=VER_STRING_GOES_HERE
  Delay1 : xbsIndex_r4/Delay  en=off  latency=3  dbl_ovrd=off  reg_retiming=off  block_type=delay
      settings: infoedit="Delay line having  configurable length.<P><P>Hardware notes: A delay line is a chain, each link of which is an SRL16 followed by a flip-flop. If register retiming is enabled, the delay line is a chain of flip-flops."  xl_area=[8 16 0 16 0 0 0]  block_version=VER_STRING_GOES_HERE
  Delay19 : xbsIndex_r4/Delay  en=off  latency=6  dbl_ovrd=off  reg_retiming=off  block_type=delay
      settings: infoedit="Delay line having  configurable length.<P><P>Hardware notes: A delay line is a chain, each link of which is an SRL16 followed by a flip-flop. If register retiming is enabled, the delay line is a chain of flip-flops."  xl_area=[9 18 0 18 0 0 0]  block_version=VER_STRING_GOES_HERE
  Delay20 : xbsIndex_r4/Delay  en=off  latency=6  dbl_ovrd=off  reg_retiming=off  block_type=delay
      settings: infoedit="Delay line having  configurable length.<P><P>Hardware notes: A delay line is a chain, each link of which is an SRL16 followed by a flip-flop. If register retiming is enabled, the delay line is a chain of flip-flops."  xl_area=[9 18 0 18 0 0 0]  block_version=VER_STRING_GOES_HERE
  Delay3 : xbsIndex_r4/Delay  en=off  latency=3  dbl_ovrd=off  reg_retiming=off  block_type=delay
      settings: infoedit="Delay line having  configurable length.<P><P>Hardware notes: A delay line is a chain, each link of which is an SRL16 followed by a flip-flop. If register retiming is enabled, the delay line is a chain of flip-flops."  xl_area=[8 16 0 16 0 0 0]  block_version=VER_STRING_GOES_HERE
  RVM0 : xbsIndex_r4/Addressable Shift Register  infer_latency=off  depth=4  initVector=[0]  en=off  dbl_ovrd=off  use_behavioral_HDL=off  use_rpm=off  block_type=addrsr
      settings: infoedit="Delay of configurable length.  Any element in the delay line can be addressed and driven onto the output port.<P><P>Hardware notes: Implemented using SRL16s.  If a Virtex-II device is used, multiple SRLC16s are cascaded together."  xl_area=[8 0 0 16 0 0 0]  block_version=VER_STRING_GOES_HERE
  RVM1 : xbsIndex_r4/Addressable Shift Register  infer_latency=off  depth=4  initVector=[0]  en=off  dbl_ovrd=off  use_behavioral_HDL=off  use_rpm=off  block_type=addrsr
      settings: infoedit="Delay of configurable length.  Any element in the delay line can be addressed and driven onto the output port.<P><P>Hardware notes: Implemented using SRL16s.  If a Virtex-II device is used, multiple SRLC16s are cascaded together."  xl_area=[8 0 0 16 0 0 0]  block_version=VER_STRING_GOES_HERE
  Up Sample : xbsIndex_r4/Up Sample  sample_ratio=4  copy_samples=on  en=off  latency=0  dbl_ovrd=off  block_type=usamp
      settings: infoedit="Up samples input data.  Inserted values  can be zeros or copies of the most recent input sample.<P><P>Hardware notes: No hardware is needed if inserted values are copies of the input sample; otherwise, a mux and single bit flip-flop are used."  xl_area=[0 0 0 0 0 0 0]  block_version=VER_STRING_GOES_HERE
  Up Sample1 : xbsIndex_r4/Up Sample  sample_ratio=4  copy_samples=on  en=off  latency=0  dbl_ovrd=off  block_type=usamp
      settings: infoedit="Up samples input data.  Inserted values  can be zeros or copies of the most recent input sample.<P><P>Hardware notes: No hardware is needed if inserted values are copies of the input sample; otherwise, a mux and single bit flip-flop are used."  xl_area=[0 0 0 0 0 0 0]  block_version=VER_STRING_GOES_HERE
  a1 : xbsIndex_r4/AddSub  mode=Addition  use_carryin=off  use_carryout=off  en=off  latency=0  precision=User Defined  arith_type="Signed  (2's comp)"  n_bits=lms_acc_ni  bin_pt=lms_acc_nf  quantization="Round  (unbiased: +/- Inf)"  overflow=Wrap  dbl_ovrd=off  use_behavioral_HDL=on  hw_selection=Fabric  pipelined=off  use_rpm=on  block_type=addsub
      settings: xl_area=[18 0 0 36 0 0 0]  block_version=VER_STRING_GOES_HERE
  a2 : xbsIndex_r4/AddSub  mode=Addition  use_carryin=off  use_carryout=off  en=off  latency=0  precision=User Defined  arith_type="Signed  (2's comp)"  n_bits=lms_acc_ni  bin_pt=lms_acc_nf  quantization="Round  (unbiased: +/- Inf)"  overflow=Wrap  dbl_ovrd=off  use_behavioral_HDL=on  hw_selection=Fabric  pipelined=off  use_rpm=on  block_type=addsub
      settings: xl_area=[18 0 0 36 0 0 0]  block_version=VER_STRING_GOES_HERE
  c3 : xbsIndex_r4/Convert  arith_type="Signed  (2's comp)"  n_bits=coeff_ni  bin_pt=coeff_nf  quantization="Round  (unbiased: +/- Inf)"  overflow=Wrap  latency=0  dbl_ovrd=off  pipeline=off  block_type=convert
      settings: infoedit=The input is presented at the output after quantization and overflow effects.<P><P>Hardware notes: Additional hardware is used when rounding or saturation is selected and output width is less than the input width.  xl_area=[11 0 0 22 0 0 0]  block_version=VER_STRING_GOES_HERE
  c4 : xbsIndex_r4/Convert  arith_type="Signed  (2's comp)"  n_bits=coeff_ni  bin_pt=coeff_nf  quantization="Round  (unbiased: +/- Inf)"  overflow=Wrap  latency=0  dbl_ovrd=off  pipeline=off  block_type=convert
      settings: infoedit=The input is presented at the output after quantization and overflow effects.<P><P>Hardware notes: Additional hardware is used when rounding or saturation is selected and output width is less than the input width.  xl_area=[11 0 0 22 0 0 0]  block_version=VER_STRING_GOES_HERE
  coef_r : Outport  OutDataType=sfix(16)  OutScaling=2^0
  coef_i : Outport  Port=2  OutDataType=sfix(16)  OutScaling=2^0
  wires:
  x_I/1 -> RVM0/1
  RVM0/1 -> Delay3/1
  x_Q/1 -> RVM1/1
  RVM1/1 -> Delay1/1
  Delay3/1 -> Cmplx Mult/1(a_r)
  Delay1/1 -> Cmplx Mult/2(a_i)
  a1/1 -> Coeff Buffer2/1(In)
  a2/1 -> Coeff Buffer1/1(In)
  Coeff Buffer2/1(Out) -> c3/1, a1/2
  Coeff Buffer1/1(Out) -> c4/1, a2/2
  err_r/1 -> Up Sample/1
  err_i/1 -> Up Sample1/1
  Up Sample/1 -> Cmplx Mult/3(b_r)
  Up Sample1/1 -> Cmplx Mult/4(b_i)
  Data Addr  Gen/1 -> Delay/1
  Delay/1 -> RVM1/2, RVM0/2
  c3/1 -> Delay20/1
  c4/1 -> Delay19/1
  Delay19/1 -> coef_i/1
  Delay20/1 -> coef_r/1
  Cmplx Mult/1(p_r) -> a1/1
  Cmplx Mult/2(p_i) -> a2/1
